simulink model "CessnaCitationCitationIIModel550_3DOF_control"  (R2020b)
settings: Solver=ode45  StartTime=0.0  StopTime=inf  FixedStep=1e-14  RelTol=1e-3
PreLoadFcn:
  | CessnaCitationData
  | datcom_data = datcomimport('Citation.out'); %Datcom data structures
  | datcom_data = FixDatcomData(datcom_data{3});
InitFcn:
  | CessnaCitationData
values from neighbouring files (symbols this model uses):
  gnd_alt = -1500    [CessnaCitationData.m]
  inertia = [19990.488, -0.000, 7138.962 ... (first row only)    [CessnaCitationData.m]
  initpos_e = [0 0 -1500]    [CessnaCitationData.m]
  initrotrates_e = [0 0 0]    [CessnaCitationData.m]
  initrpy_e = [0 0 0]    [CessnaCitationData.m]
  initvel_b = [85 0 0]    [CessnaCitationData.m]
  K = [-1.67126776797  253.63980268  1.10078856748  -2.4851948262  39.0629348129; 35.3806265678  -3943.84542644  -7.5960479952  17.7911501004  203.328962985]    [state_feedback_gain.mat]
  mass = 3175    [CessnaCitationData.m]
  max_thrust = 1134    [CessnaCitationData.m]
  wind_angle_rates = [0 0 0]    [CessnaCitationData.m]
undefined symbols (not defined in the file or in its folder): Earth, WGS84
libraries: aerolibtransform2 x5, aerolibasang x4, aerolibadyn x2, aerolibanim x1, aerolibwind2 x1, aerolibatmos2 x1, shared3dof x1, sharedtransform x1, simulink_extras x1
settings Model: Creator=pasquale  LastModifiedBy=pasquale
settings DataIOCC: ExternalInput=getinputstruct(op_trim1)  InitialState=getstatestruct(op_trim1)

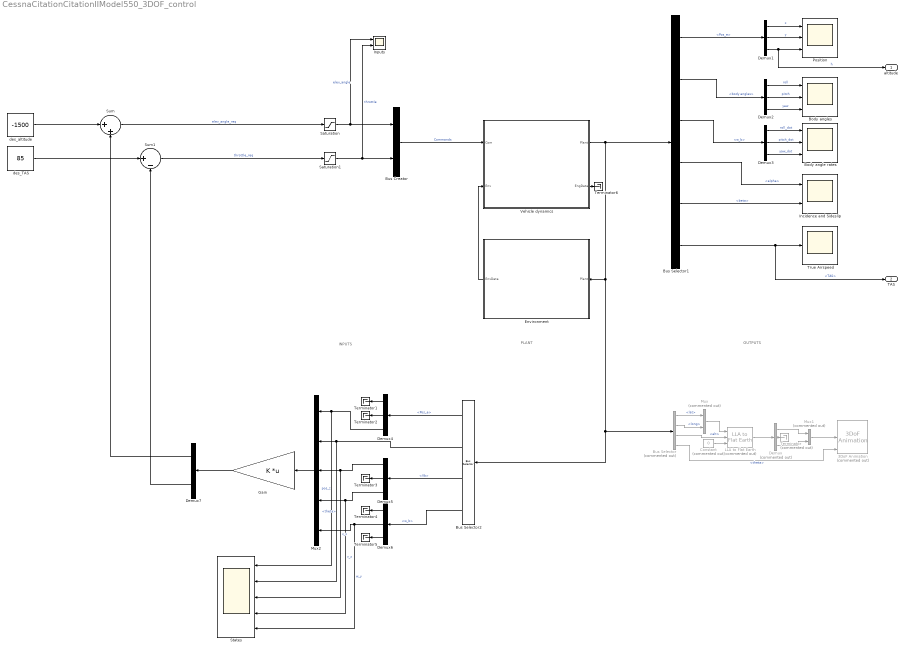
== system CessnaCitationCitationIIModel550_3DOF_control ==
  note: OUTPUTS
  note: PLANT
  note: INPUTS
  3DoF Animation : aerolibanim/3DoF Animation  Commented=on  u1=[0 5000 -2000 2000 -5050 -3050]  u2=0.05  u3=1.0  u5=Fixed position  u6=[2000 500 -3150]  u7=10  u8=on
      settings: SourceProductBaseCode=AE
  Body angle rates : Scope  NumInputPorts=3
  Body angles : Scope  NumInputPorts=3
  Bus Creator : BusCreator  Inputs=2
  Bus Selector : BusSelector  Commented=on  OutputSignals=lat,long,alt,body angles.theta
  Bus Selector1 : BusSelector  OutputSignals=Pos_e,body angles,w_b,alpha,beta,TAS
  Bus Selector2 : BusSelector  OutputSignals=Pos_e,body angles.theta,Vb,w_b
  Constant : Constant  Commented=on  Value=0
  Demux : Demux  Commented=on  Outputs=3
  Demux{1..6} (6 alike) : Demux  Outputs=3
  Demux7 : Demux  Outputs=2
  Environment : Subsystem
      mask Display: image('521928855-56a132c45f9b58b7d0bcf732-1.jpg'); % Use "Edit Image" on toolstrip to change.
  Gain : Gain  Gain=K  Multiplication=Matrix(K*u)
  Incidence and Sideslip : Scope  NumInputPorts=2
  Inputs : Scope  NumInputPorts=2
  LLA to Flat Earth : aerolibtransform2/LLA to Flat Earth  Commented=on  units=Metric (MKS)  ptype=Earth (WGS84)  F=1/298.257223563  R=6378137  refPosPort=off  LL0=[0 10]  psi=0
      settings: SourceProductBaseCode=AE
  Mux : Mux  Commented=on  Inputs=2
  Mux1 : Mux  Commented=on  Inputs=2
  Mux2 : Mux  Inputs=5
  Position : Scope  NumInputPorts=3
  Saturation : Saturate  UpperLimit=20  LowerLimit=-20
  Saturation1 : Saturate  UpperLimit=10000  LowerLimit=0
  States : Scope  NumInputPorts=5
  Sum : Sum  Inputs=|++
  Sum1 : Sum  Inputs=|+-
  Terminator : Terminator  Commented=on
  Terminator{1..6} (6 alike) : Terminator
  True Airspeed : Scope
  Vehicle dynamics : Subsystem
      mask Display: image('Cessna-Citation-II-IISP-S.jpg'); % Use "Edit Image" on toolstrip to change.
  des_TAS : Constant  Value=85
  des_altitude : Constant  Value=-1500
  altitude : Outport
  TAS : Outport  Port=2
  wires:
  Environment/1(EnvData) -> Vehicle dynamics/2(Env)
  Constant/1 -> LLA to Flat Earth/3
  Bus Selector/1 -> Mux/1  "<lat>"
  Bus Selector/2 -> Mux/2  "<long>"
  Mux/1 -> LLA to Flat Earth/1
  Bus Selector/3 -> LLA to Flat Earth/2  "<alt>"
  Bus Selector/4 -> 3DoF Animation/3  "<theta>"
  LLA to Flat Earth/1 -> Demux/1
  Demux/1 -> Mux1/1
  Demux/3 -> Mux1/2
  Demux/2 -> Terminator/1
  Mux1/1 -> 3DoF Animation/2
  Vehicle dynamics/1(Plant) -> Environment/1(Plant), Bus Selector2/1, Bus Selector/1, Bus Selector1/1
  Bus Creator/1 -> Vehicle dynamics/1(Com)  "Commands"
  Bus Selector1/1 -> Demux1/1  "<Pos_e>"
  Demux1/1 -> Position/1  "x"
  Demux1/2 -> Position/2  "y"
  Demux1/3 -> Position/3, altitude/1  "h"
  Bus Selector1/2 -> Demux2/1  "<body angles>"
  Demux2/1 -> Body angles/1  "roll"
  Demux2/2 -> Body angles/2  "pitch"
  Demux2/3 -> Body angles/3  "yaw"
  Bus Selector1/3 -> Demux3/1  "<w_b>"
  Demux3/1 -> Body angle rates/1  "roll_dot"
  Demux3/2 -> Body angle rates/2  "pitch_dot"
  Demux3/3 -> Body angle rates/3  "yaw_dot"
  Bus Selector1/4 -> Incidence and Sideslip/1  "<alpha>"
  Bus Selector1/5 -> Incidence and Sideslip/2  "<beta>"
  Bus Selector1/6 -> TAS/1, True Airspeed/1  "<TAS>"
  Bus Selector2/1 -> Demux4/1  "<Pos_e>"
  Bus Selector2/2 -> States/2, Mux2/2  "<theta>"
  Bus Selector2/3 -> Demux5/1  "<Vb>"
  Bus Selector2/4 -> Demux6/1  "<w_b>"
  Demux4/3 -> States/1, Mux2/1  "pos_z"
  Demux5/1 -> States/3, Mux2/3  "v_x"
  Demux6/2 -> States/5, Mux2/5  "w_y"
  Demux4/1 -> Terminator1/1
  Demux6/3 -> Terminator5/1
  Demux6/1 -> Terminator4/1
  Demux5/2 -> Terminator3/1
  Demux4/2 -> Terminator2/1
  Demux7/1 -> Sum/2
  Demux7/2 -> Sum1/2
  des_altitude/1 -> Sum/1
  des_TAS/1 -> Sum1/1
  Sum/1 -> Saturation/1  "elev_angle_req"
  Sum1/1 -> Saturation1/1  "throttle_req"
  Vehicle dynamics/2(EngData) -> Terminator6/1
  Saturation/1 -> Inputs/1, Bus Creator/1  "elev_angle"
  Saturation1/1 -> Inputs/2, Bus Creator/2  "throttle"
  Demux5/3 -> States/4, Mux2/4  "v_z"
  Mux2/1 -> Gain/1
  Gain/1 -> Demux7/1

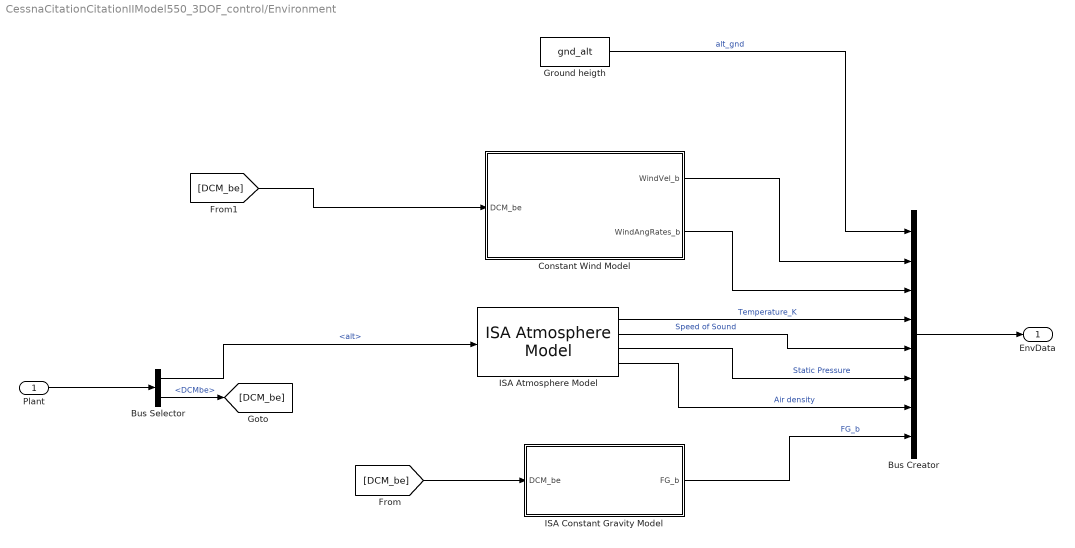
== system CessnaCitationCitationIIModel550_3DOF_control/Environment ==
  Plant : Inport
  Bus Creator : BusCreator  Inputs=8
  Bus Selector : BusSelector  OutputSignals=alt,DCMbe
  Constant Wind Model : Subsystem
  Ground heigth : Constant  Value=gnd_alt
  ISA Atmosphere Model : aerolibatmos2/ISA Atmosphere Model  custom=off  g=9.80665  gamma=1.4  R=287.0531  L=0.0065  h_trop=11000  h_strat=20000  rho0=1.225  P0=101325  T0=288.15  h0=0
  ISA Constant Gravity Model : Subsystem
  EnvData : Outport
  wires:
  Plant/1 -> Bus Selector/1
  Bus Selector/1 -> ISA Atmosphere Model/1  "<alt>"
  Bus Creator/1 -> EnvData/1
  ISA Atmosphere Model/4 -> Bus Creator/7  "Air density"
  ISA Atmosphere Model/3 -> Bus Creator/6  "Static Pressure"
  ISA Atmosphere Model/2 -> Bus Creator/5  "Speed of Sound"
  ISA Atmosphere Model/1 -> Bus Creator/4  "Temperature_K"
  Bus Selector/2 -> [DCM_be]  "<DCMbe>"
  [DCM_be] -> Constant Wind Model/1(DCM_be)
  Constant Wind Model/1(WindVel_b) -> Bus Creator/2
  Constant Wind Model/2(WindAngRates_b) -> Bus Creator/3
  ISA Constant Gravity Model/1(FG_b) -> Bus Creator/8  "FG_b"
  [DCM_be] -> ISA Constant Gravity Model/1(DCM_be)
  Ground heigth/1 -> Bus Creator/1  "alt_gnd"

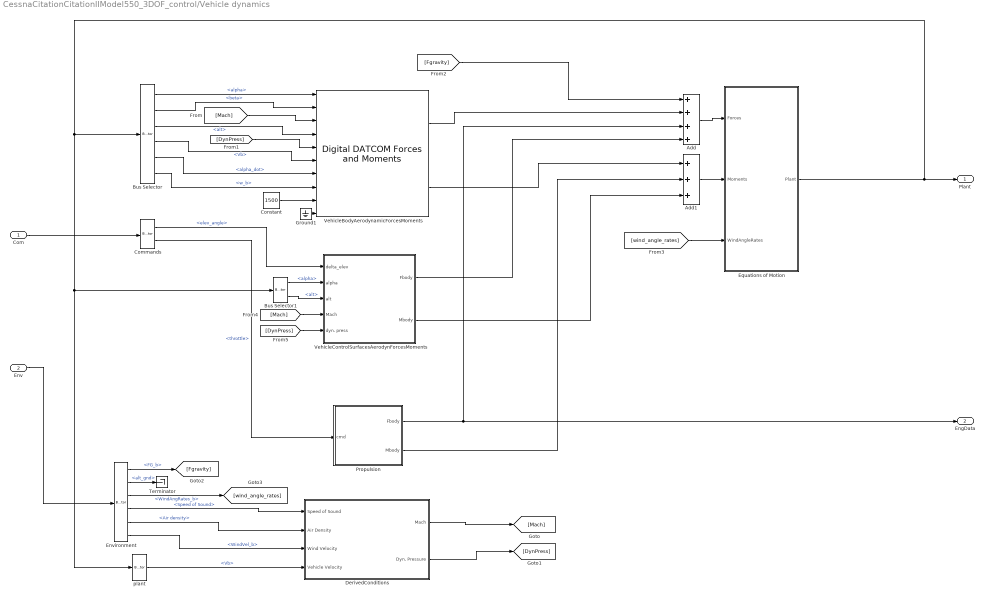
== system CessnaCitationCitationIIModel550_3DOF_control/Vehicle dynamics ==
  Com : Inport
  Env : Inport  Port=2
  Add : Sum  Inputs=++++
  Add1 : Sum  Inputs=+++
  Bus Selector : BusSelector  OutputSignals=alpha,beta,alt,Vb,alpha_dot,w_b
  Bus Selector1 : BusSelector  OutputSignals=alpha,alt
  Commands : BusSelector  OutputSignals=elev_angle,throttle
  Constant : Constant  Value=1500
  DerivedConditions : Subsystem
  Environment : BusSelector  OutputSignals=FG_b,alt_gnd,WindAngRates_b,Speed of Sound,Air density,WindVel_b
  Equations of Motion : Subsystem
  Ground1 : Ground
  Propulsion : Subsystem
  Terminator : Terminator
  VehicleBodyAerodynamicForcesMoments : aerolibadyn/Digital DATCOM Forces and Moments  units=Metric (MKS)  dcase=datcom_data  fmode=Body  buildno=0  imethod=Linear  emethod=Linear  rmethod=Linear Extrapolation  action=None
      settings: SourceProductBaseCode=AE
  VehicleControlSurfacesAerodynForcesMoments : Subsystem
  plant : BusSelector  OutputSignals=Vb
  Plant : Outport
  EngData : Outport  Port=2
  wires:
  Propulsion/1(Fbody) -> Add/3, EngData/1
  DerivedConditions/2(Dyn. Pressure) -> [DynPress]
  DerivedConditions/1(Mach) -> [Mach]
  [Mach] -> VehicleBodyAerodynamicForcesMoments/3
  [DynPress] -> VehicleBodyAerodynamicForcesMoments/5
  Bus Selector/2 -> VehicleBodyAerodynamicForcesMoments/2  "<beta>"
  Bus Selector/3 -> VehicleBodyAerodynamicForcesMoments/4  "<alt>"
  Bus Selector/4 -> VehicleBodyAerodynamicForcesMoments/6  "<Vb>"
  Bus Selector/6 -> VehicleBodyAerodynamicForcesMoments/8  "<w_b>"
  plant/1 -> DerivedConditions/4(Vehicle Velocity)  "<Vb>"
  Equations of Motion/1(Plant) -> plant/1, Bus Selector1/1, Bus Selector/1, Plant/1
  Env/1 -> Environment/1
  Com/1 -> Commands/1
  Environment/6 -> DerivedConditions/3(Wind Velocity)  "<WindVel_b>"
  Environment/5 -> DerivedConditions/2(Air Density)  "<Air density>"
  Environment/4 -> DerivedConditions/1(Speed of Sound)  "<Speed of Sound>"
  Commands/2 -> Propulsion/1(cmd)  "<throttle>"
  Bus Selector/1 -> VehicleBodyAerodynamicForcesMoments/1  "<alpha>"
  Bus Selector/5 -> VehicleBodyAerodynamicForcesMoments/7  "<alpha_dot>"
  Commands/1 -> VehicleControlSurfacesAerodynForcesMoments/1(delta_elev)  "<elev_angle>"
  Environment/1 -> [Fgravity]  "<FG_b>"
  Environment/3 -> [wind_angle_rates]  "<WindAngRates_b>"
  [wind_angle_rates] -> Equations of Motion/3(WindAngleRates)
  [Fgravity] -> Add/1
  VehicleBodyAerodynamicForcesMoments/1 -> Add/2
  VehicleBodyAerodynamicForcesMoments/2 -> Add1/1
  Propulsion/2(Mbody) -> Add1/2
  Add/1 -> Equations of Motion/1(Forces)
  Add1/1 -> Equations of Motion/2(Moments)
  VehicleControlSurfacesAerodynForcesMoments/1(Fbody) -> Add/4
  VehicleControlSurfacesAerodynForcesMoments/2(Mbody) -> Add1/3
  Bus Selector1/1 -> VehicleControlSurfacesAerodynForcesMoments/2(alpha)  "<alpha>"
  Bus Selector1/2 -> VehicleControlSurfacesAerodynForcesMoments/3(alt)  "<alt>"
  [DynPress] -> VehicleControlSurfacesAerodynForcesMoments/5(dyn. press)
  [Mach] -> VehicleControlSurfacesAerodynForcesMoments/4(Mach)
  Constant/1 -> VehicleBodyAerodynamicForcesMoments/9
  Ground1/1 -> VehicleBodyAerodynamicForcesMoments/10
  Environment/2 -> Terminator/1  "<alt_gnd>"

== system CessnaCitationCitationIIModel550_3DOF_control/Environment/Constant Wind Model ==
  DCM_be : Inport
  Horizontal Wind Model : aerolibwind2/Horizontal Wind Model  units=Metric (MKS)  Vw_source=Internal  Vwind=wind_speed  W_source=Internal  Wdeg=wind_dir
      settings: SourceProductBaseCode=AE
  Product2 : Product  Multiplication=Matrix(*)
  Wind_ang_rates : Constant  Value=wind_angle_rates
  WindVel_b : Outport
  WindAngRates_b : Outport  Port=2
  wires:
  DCM_be/1 -> Horizontal Wind Model/1, Product2/1
  Horizontal Wind Model/1 -> WindVel_b/1  "WindVel_b"
  Wind_ang_rates/1 -> Product2/2
  Product2/1 -> WindAngRates_b/1  "WindAngRates_b"

== system CessnaCitationCitationIIModel550_3DOF_control/Environment/ISA Constant Gravity Model ==
  DCM_be : Inport
  Gain : Gain  Gain=[0 0 mass]
  ISA constant gravity : Constant  Value=9.80665
  Product : Product  Multiplication=Matrix(*)
  FG_b : Outport
  wires:
  ISA constant gravity/1 -> Gain/1
  Gain/1 -> Product/2  "Fg in flat earth axis"
  DCM_be/1 -> Product/1
  Product/1 -> FG_b/1  "FG_b"

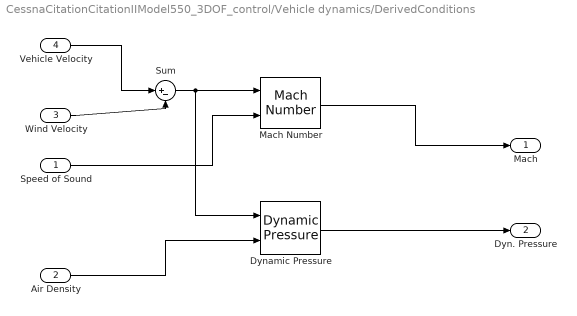
== system CessnaCitationCitationIIModel550_3DOF_control/Vehicle dynamics/DerivedConditions ==
  Speed of Sound : Inport
  Air Density : Inport  Port=2
  Wind Velocity : Inport  Port=3
  Vehicle Velocity : Inport  Port=4
  Dynamic Pressure : aerolibasang/Dynamic Pressure
  Mach Number : aerolibasang/Mach Number
      settings: SourceProductBaseCode=AE
  Sum : Sum  Inputs=|+-
  Mach : Outport
  Dyn. Pressure : Outport  Port=2
  wires:
  Vehicle Velocity/1 -> Sum/1
  Wind Velocity/1 -> Sum/2
  Sum/1 -> Dynamic Pressure/1, Mach Number/1
  Speed of Sound/1 -> Mach Number/2
  Mach Number/1 -> Mach/1
  Dynamic Pressure/1 -> Dyn. Pressure/1
  Air Density/1 -> Dynamic Pressure/2

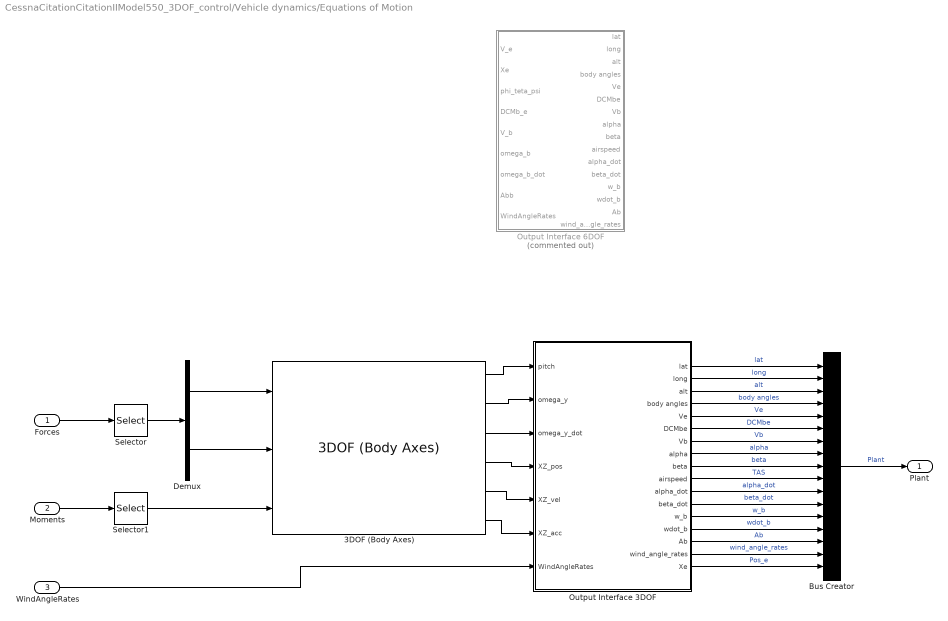
== system CessnaCitationCitationIIModel550_3DOF_control/Vehicle dynamics/Equations of Motion ==
  Forces : Inport
  Moments : Inport  Port=2
  WindAngleRates : Inport  Port=3
  3DOF (Body Axes) : shared3dof/3DOF (Body Axes)  units=Metric (MKS)  mtype=Fixed  v_ini=initvel_b(1)  theta_ini=initrpy_e(2)  alpha_ini=0  pos_ini=[initpos_e(1) initpos_e(3)]  q_ini=initrotrates_e(2)  mass=mass  mass_e=0.5  mass_f=3.0  Iyy=inertia(2,2)  Iyy_e=0.5  Iyy_f=3.0  g_in=Internal  g=0  vre_flag=on  abi_flag=off  aMode=0  vel_statename=''  theta_statename=''  pos_statename=''  q_statename=''  mass_statename=''
      settings: SourceProductBaseCode=AE,PW,MT,UV,VE,VP
  Bus Creator : BusCreator  Inputs=17
  Demux : Demux  Outputs=2
  Output Interface 3DOF : Subsystem
  Output Interface 6DOF : Subsystem  Commented=on
  Selector : Selector  InputPortWidth=3  IndexOptions=Index vector (dialog)  Indices=[1 3]  OutputSizes=1
  Selector1 : Selector  InputPortWidth=3  IndexOptions=Index vector (dialog)  Indices=[2]  OutputSizes=1
  Plant : Outport
  wires:
  Bus Creator/1 -> Plant/1  "Plant"
  Forces/1 -> Selector/1
  Demux/1 -> 3DOF (Body Axes)/1
  Demux/2 -> 3DOF (Body Axes)/2
  Selector/1 -> Demux/1
  Moments/1 -> Selector1/1
  Selector1/1 -> 3DOF (Body Axes)/3
  3DOF (Body Axes)/3 -> Output Interface 3DOF/3(omega_y_dot)
  3DOF (Body Axes)/1 -> Output Interface 3DOF/1(pitch)
  3DOF (Body Axes)/2 -> Output Interface 3DOF/2(omega_y)
  3DOF (Body Axes)/4 -> Output Interface 3DOF/4(XZ_pos)
  3DOF (Body Axes)/5 -> Output Interface 3DOF/5(XZ_vel)
  3DOF (Body Axes)/6 -> Output Interface 3DOF/6(XZ_acc)
  Output Interface 3DOF/1(lat) -> Bus Creator/1  "lat"
  Output Interface 3DOF/2(long) -> Bus Creator/2  "long"
  Output Interface 3DOF/3(alt) -> Bus Creator/3  "alt"
  Output Interface 3DOF/4(body angles) -> Bus Creator/4  "body angles"
  Output Interface 3DOF/5(Ve) -> Bus Creator/5  "Ve"
  Output Interface 3DOF/6(DCMbe) -> Bus Creator/6  "DCMbe"
  Output Interface 3DOF/7(Vb) -> Bus Creator/7  "Vb"
  Output Interface 3DOF/8(alpha) -> Bus Creator/8  "alpha"
  Output Interface 3DOF/9(beta) -> Bus Creator/9  "beta"
  Output Interface 3DOF/10(airspeed) -> Bus Creator/10  "TAS"
  Output Interface 3DOF/11(alpha_dot) -> Bus Creator/11  "alpha_dot"
  Output Interface 3DOF/12(beta_dot) -> Bus Creator/12  "beta_dot"
  Output Interface 3DOF/13(w_b) -> Bus Creator/13  "w_b"
  Output Interface 3DOF/14(wdot_b) -> Bus Creator/14  "wdot_b"
  Output Interface 3DOF/15(Ab) -> Bus Creator/15  "Ab"
  Output Interface 3DOF/16(wind_angle_rates) -> Bus Creator/16  "wind_angle_rates"
  WindAngleRates/1 -> Output Interface 3DOF/7(WindAngleRates)
  Output Interface 3DOF/17(Xe) -> Bus Creator/17  "Pos_e"

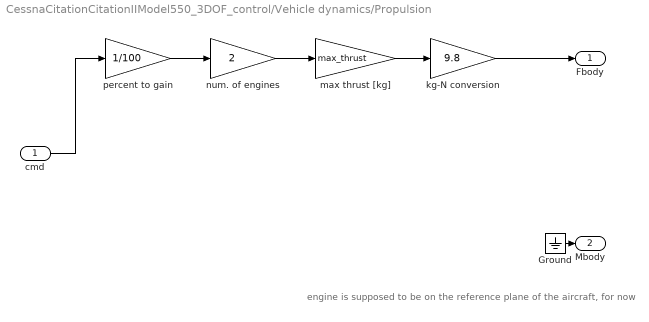
== system CessnaCitationCitationIIModel550_3DOF_control/Vehicle dynamics/Propulsion ==
  note: engine is supposed to be on the reference plane of the aircraft, for now
  cmd : Inport
  Ground : Ground
  kg-N conversion : Gain  Gain=9.8
  max thrust [kg] : Gain  Gain=max_thrust
  num. of engines : Gain  Gain=2
  percent to gain : Gain  Gain=1/100
  Fbody : Outport
  Mbody : Outport  Port=2
  wires:
  percent to gain/1 -> num. of engines/1
  cmd/1 -> percent to gain/1
  max thrust [kg]/1 -> kg-N conversion/1
  kg-N conversion/1 -> Fbody/1
  Ground/1 -> Mbody/1
  num. of engines/1 -> max thrust [kg]/1

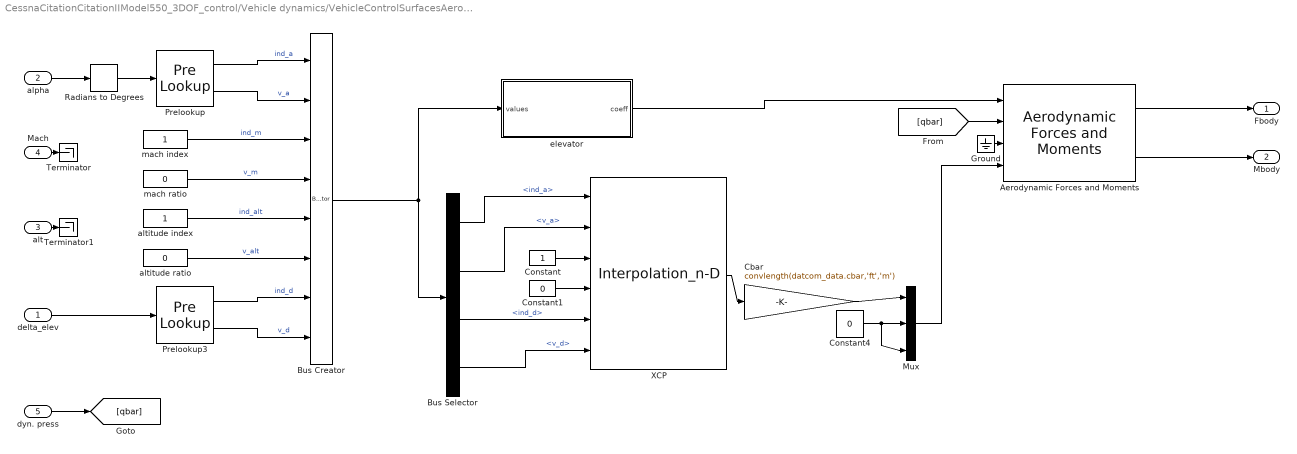
== system CessnaCitationCitationIIModel550_3DOF_control/Vehicle dynamics/VehicleControlSurfacesAerodynForcesMoments ==
  delta_elev : Inport
  alpha : Inport  Port=2
  alt : Inport  Port=3
  Mach : Inport  Port=4
  dyn. press : Inport  Port=5
  "Aerodynamic Forces and Moments " : aerolibadyn/Aerodynamic Forces and Moments   inputAxes=Body  outputForceAxes=Body  outputMomentAxes=Body  S=convlength(datcom_data.sref,'ft','m')  b=convlength(datcom_data.blref,'ft','m')  cbar=convlength(datcom_data.cbar,'ft','m')
  Bus Creator : BusCreator  Inputs=8
  Bus Selector : BusSelector  OutputSignals=ind_a,v_a,ind_d,v_d
  Cbar : Gain  Gain=convlength(datcom_data.cbar,'ft','m')
  Constant : Constant
  Constant1 : Constant  Value=0
  Constant4 : Constant  Value=0
  Ground : Ground
  Mux : Mux  Inputs=3
  Prelookup : PreLookup  BreakpointsData=datcom_data.alpha  ExtrapMethod=Linear
  Prelookup3 : PreLookup  BreakpointsData=datcom_data.delta  ExtrapMethod=Linear
  Radians to Degrees : simulink_extras/Transformations/Radians to Degrees
  Terminator : Terminator
  Terminator1 : Terminator
  XCP : Interpolation_n-D  NumberOfTableDimensions=3  Table=reshape(datcom_data.xcp, [20 2 9]);  InternalRulePriority=Speed
      settings: InputPortMap=u0,u1,u2,u3,u4,u5
  altitude index : Constant
  altitude ratio : Constant  Value=0
  elevator : Subsystem
  mach index : Constant
  mach ratio : Constant  Value=0
  Fbody : Outport
  Mbody : Outport  Port=2
  wires:
  alpha/1 -> Radians to Degrees/1
  Radians to Degrees/1 -> Prelookup/1
  delta_elev/1 -> Prelookup3/1
  Prelookup/1 -> Bus Creator/1  "ind_a"
  Prelookup/2 -> Bus Creator/2  "v_a"
  Prelookup3/1 -> Bus Creator/7  "ind_d"
  Prelookup3/2 -> Bus Creator/8  "v_d"
  Bus Creator/1 -> elevator/1(values), Bus Selector/1
  Mach/1 -> Terminator/1
  alt/1 -> Terminator1/1
  mach index/1 -> Bus Creator/3  "ind_m"
  mach ratio/1 -> Bus Creator/4  "v_m"
  altitude index/1 -> Bus Creator/5  "ind_alt"
  altitude ratio/1 -> Bus Creator/6  "v_alt"
  dyn. press/1 -> [qbar]
  [qbar] -> "Aerodynamic Forces and Moments "/2
  Ground/1 -> "Aerodynamic Forces and Moments "/3
  elevator/1(coeff) -> "Aerodynamic Forces and Moments "/1
  Bus Selector/1 -> XCP/1  "<ind_a>"
  Bus Selector/2 -> XCP/2  "<v_a>"
  Constant1/1 -> XCP/4
  Constant/1 -> XCP/3
  Bus Selector/3 -> XCP/5  "<ind_d>"
  Bus Selector/4 -> XCP/6  "<v_d>"
  XCP/1 -> Cbar/1
  Constant4/1 -> Mux/3, Mux/2
  Mux/1 -> "Aerodynamic Forces and Moments "/4
  "Aerodynamic Forces and Moments "/1 -> Fbody/1
  "Aerodynamic Forces and Moments "/2 -> Mbody/1
  Cbar/1 -> Mux/1

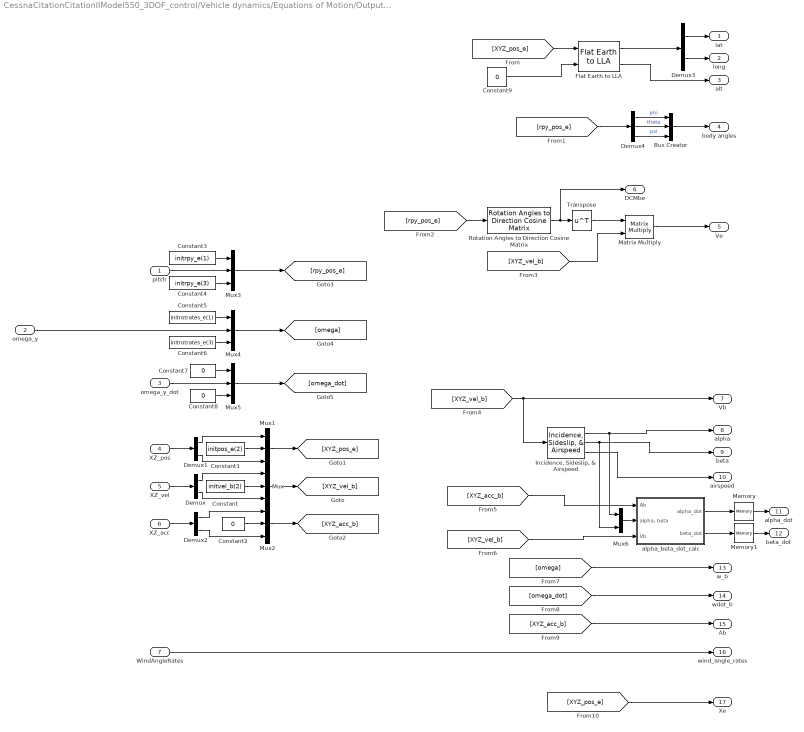
== system CessnaCitationCitationIIModel550_3DOF_control/Vehicle dynamics/Equations of Motion/Output Interface 3DOF ==
  pitch : Inport
  omega_y : Inport  Port=2
  omega_y_dot : Inport  Port=3
  XZ_pos : Inport  Port=4
  XZ_vel : Inport  Port=5
  XZ_acc : Inport  Port=6
  WindAngleRates : Inport  Port=7
  Bus Creator : BusCreator  Inputs=3
  Constant : Constant  Value=initvel_b(2)
  Constant1 : Constant  Value=initpos_e(2)
  Constant{2,7..9} (4 alike) : Constant  Value=0
  Constant3 : Constant  Value=initrpy_e(1)
  Constant4 : Constant  Value=initrpy_e(3)
  Constant5 : Constant  Value=initrotrates_e(1)
  Constant6 : Constant  Value=initrotrates_e(3)
  Demux{,1..3} (4 alike) : Demux  Outputs=2
  Demux4 : Demux  Outputs=3
  Flat Earth to LLA : aerolibtransform2/Flat Earth to LLA  units=Metric (MKS)  ptype=Earth (WGS84)  F=1/298.257223563  R=6378137  refPosPort=off  LL0=[0 10]  psi=0
  "Incidence, Sideslip, & Airspeed" : aerolibasang/Incidence, Sideslip, & Airspeed
  Matrix Multiply : Product  Multiplication=Matrix(*)
  Memory : Memory
  Memory1 : Memory
  Mux{,1..5} (6 alike) : Mux  Inputs=3
  Mux6 : Mux  Inputs=2
  Rotation Angles to Direction Cosine Matrix : sharedtransform/Rotation Angles to Direction Cosine Matrix  rotationOrder=ZYX  aMode=aMode
      settings: SourceProductBaseCode=AE,PW,MT,UV,VE,VP
  Transpose : Math  Operator=transpose  SaturateOnIntegerOverflow=on
  alpha_beta_dot_calc : Subsystem
  lat : Outport
  long : Outport  Port=2
  alt : Outport  Port=3
  body angles : Outport  Port=4
  Ve : Outport  Port=5
  DCMbe : Outport  Port=6
  Vb : Outport  Port=7
  alpha : Outport  Port=8
  beta : Outport  Port=9
  airspeed : Outport  Port=10
  alpha_dot : Outport  Port=11
  beta_dot : Outport  Port=12
  w_b : Outport  Port=13
  wdot_b : Outport  Port=14
  Ab : Outport  Port=15
  wind_angle_rates : Outport  Port=16
  Xe : Outport  Port=17
  wires:
  WindAngleRates/1 -> wind_angle_rates/1
  XZ_vel/1 -> Demux/1
  Constant/1 -> Mux/2
  Demux/1 -> Mux/1
  Demux/2 -> Mux/3
  Mux/1 -> [XYZ_vel_b]
  Mux1/1 -> [XYZ_pos_e]
  Demux1/2 -> Mux1/3
  Demux1/1 -> Mux1/1
  Constant1/1 -> Mux1/2
  XZ_pos/1 -> Demux1/1
  Constant2/1 -> Mux2/2
  Demux2/2 -> Mux2/3
  XZ_acc/1 -> Demux2/1
  Mux2/1 -> [XYZ_acc_b]
  Demux2/1 -> Mux2/1
  pitch/1 -> Mux3/2
  Constant3/1 -> Mux3/1
  Constant4/1 -> Mux3/3
  Mux3/1 -> [rpy_pos_e]
  Mux4/1 -> [omega]
  Constant6/1 -> Mux4/3
  Constant5/1 -> Mux4/1
  omega_y/1 -> Mux4/2
  omega_y_dot/1 -> Mux5/2
  Constant7/1 -> Mux5/1
  Constant8/1 -> Mux5/3
  Mux5/1 -> [omega_dot]
  Demux3/1 -> lat/1
  Demux3/2 -> long/1
  Flat Earth to LLA/1 -> Demux3/1
  Flat Earth to LLA/2 -> alt/1
  [XYZ_pos_e] -> Flat Earth to LLA/1
  Constant9/1 -> Flat Earth to LLA/2
  Demux4/2 -> Bus Creator/2  "theta"
  Demux4/1 -> Bus Creator/1  "phi"
  Demux4/3 -> Bus Creator/3  "psi"
  Bus Creator/1 -> body angles/1
  [rpy_pos_e] -> Demux4/1
  [rpy_pos_e] -> Rotation Angles to Direction Cosine Matrix/1
  Rotation Angles to Direction Cosine Matrix/1 -> DCMbe/1, Transpose/1
  Transpose/1 -> Matrix Multiply/1
  [XYZ_vel_b] -> Matrix Multiply/2
  Matrix Multiply/1 -> Ve/1
  [XYZ_vel_b] -> "Incidence, Sideslip, & Airspeed"/1, Vb/1
  "Incidence, Sideslip, & Airspeed"/1 -> Mux6/1, alpha/1
  "Incidence, Sideslip, & Airspeed"/2 -> Mux6/2, beta/1
  "Incidence, Sideslip, & Airspeed"/3 -> airspeed/1
  Memory/1 -> alpha_dot/1
  Memory1/1 -> beta_dot/1
  [omega] -> w_b/1
  [omega_dot] -> wdot_b/1
  [XYZ_acc_b] -> Ab/1
  alpha_beta_dot_calc/1(alpha_dot) -> Memory/1
  alpha_beta_dot_calc/2(beta_dot) -> Memory1/1
  Mux6/1 -> alpha_beta_dot_calc/2("alpha, beta")
  [XYZ_acc_b] -> alpha_beta_dot_calc/1(Ab)
  [XYZ_vel_b] -> alpha_beta_dot_calc/3(Vb)
  [XYZ_pos_e] -> Xe/1

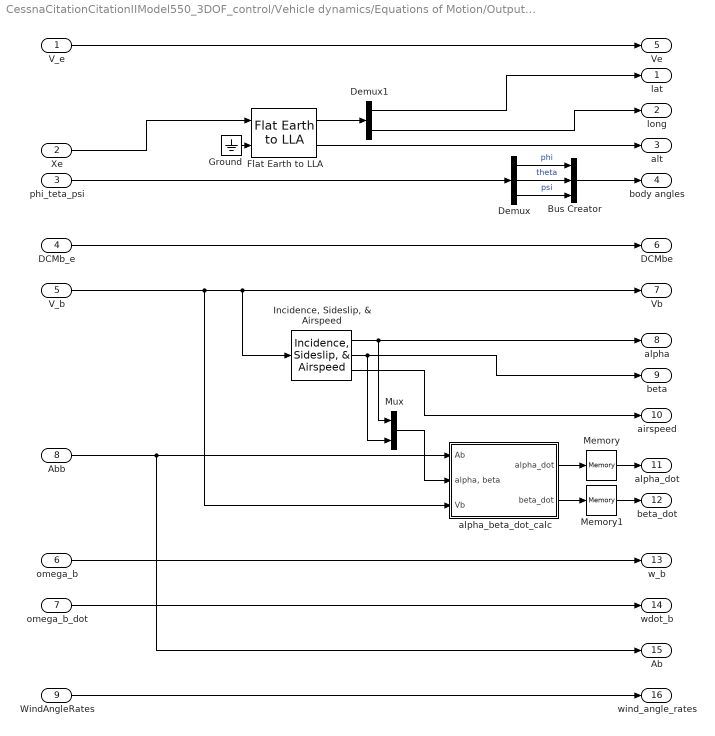
== system CessnaCitationCitationIIModel550_3DOF_control/Vehicle dynamics/Equations of Motion/Output Interface 6DOF ==
  V_e : Inport
  Xe : Inport  Port=2
  phi_teta_psi : Inport  Port=3
  DCMb_e : Inport  Port=4
  V_b : Inport  Port=5
  omega_b : Inport  Port=6
  omega_b_dot : Inport  Port=7
  Abb : Inport  Port=8
  WindAngleRates : Inport  Port=9
  Bus Creator : BusCreator  Inputs=3
  Demux : Demux  Outputs=3
  Demux1 : Demux  Outputs=2
  Flat Earth to LLA : aerolibtransform2/Flat Earth to LLA  units=Metric (MKS)  ptype=Earth (WGS84)  F=1/298.257223563  R=6378137  refPosPort=off  LL0=[0 10]  psi=0
  Ground : Ground
  "Incidence, Sideslip, & Airspeed" : aerolibasang/Incidence, Sideslip, & Airspeed
  Memory : Memory
  Memory1 : Memory
  Mux : Mux  Inputs=2
  alpha_beta_dot_calc : Subsystem
  lat : Outport
  long : Outport  Port=2
  alt : Outport  Port=3
  body angles : Outport  Port=4
  Ve : Outport  Port=5
  DCMbe : Outport  Port=6
  Vb : Outport  Port=7
  alpha : Outport  Port=8
  beta : Outport  Port=9
  airspeed : Outport  Port=10
  alpha_dot : Outport  Port=11
  beta_dot : Outport  Port=12
  w_b : Outport  Port=13
  wdot_b : Outport  Port=14
  Ab : Outport  Port=15
  wind_angle_rates : Outport  Port=16
  wires:
  Demux/2 -> Bus Creator/2  "theta"
  Ground/1 -> Flat Earth to LLA/2
  Demux/3 -> Bus Creator/3  "psi"
  Demux1/1 -> lat/1
  Flat Earth to LLA/2 -> alt/1
  Flat Earth to LLA/1 -> Demux1/1
  Demux1/2 -> long/1
  Demux/1 -> Bus Creator/1  "phi"
  Bus Creator/1 -> body angles/1
  phi_teta_psi/1 -> Demux/1
  Xe/1 -> Flat Earth to LLA/1
  DCMb_e/1 -> DCMbe/1
  V_b/1 -> alpha_beta_dot_calc/3(Vb), "Incidence, Sideslip, & Airspeed"/1, Vb/1
  "Incidence, Sideslip, & Airspeed"/1 -> Mux/1, alpha/1
  "Incidence, Sideslip, & Airspeed"/2 -> Mux/2, beta/1
  "Incidence, Sideslip, & Airspeed"/3 -> airspeed/1
  Abb/1 -> Ab/1, alpha_beta_dot_calc/1(Ab)
  Mux/1 -> alpha_beta_dot_calc/2("alpha, beta")
  V_e/1 -> Ve/1
  omega_b/1 -> w_b/1
  omega_b_dot/1 -> wdot_b/1
  WindAngleRates/1 -> wind_angle_rates/1
  alpha_beta_dot_calc/1(alpha_dot) -> Memory/1
  alpha_beta_dot_calc/2(beta_dot) -> Memory1/1
  Memory/1 -> alpha_dot/1
  Memory1/1 -> beta_dot/1

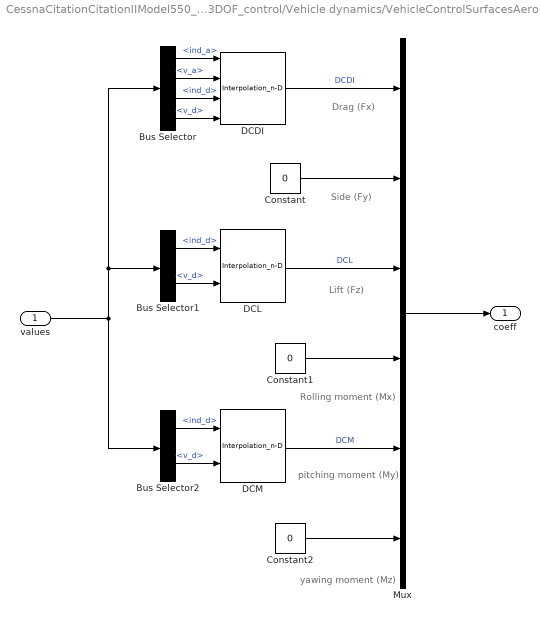
== system CessnaCitationCitationIIModel550_3DOF_control/Vehicle dynamics/VehicleControlSurfacesAerodynForcesMoments/elevator ==
  note: yawing moment (Mz)
  note: pitching moment (My)
  note: Rolling moment (Mx)
  note: Lift (Fz)
  note: Side (Fy)
  note: Drag (Fx)
  values : Inport
  Bus Selector : BusSelector  OutputSignals=ind_a,v_a,ind_d,v_d
  Bus Selector1 : BusSelector  OutputSignals=ind_d,v_d
  Bus Selector2 : BusSelector  OutputSignals=ind_d,v_d
  Constant : Constant  Value=0
  Constant1 : Constant  Value=0
  Constant2 : Constant  Value=0
  DCDI : Interpolation_n-D  Table=datcom_data.dcdi_sym  InternalRulePriority=Speed
  DCL : Interpolation_n-D  NumberOfTableDimensions=1  Table=datcom_data.dcl_sym  InternalRulePriority=Speed
      settings: InputPortMap=u0,u1
  DCM : Interpolation_n-D  NumberOfTableDimensions=1  Table=datcom_data.dcl_sym  InternalRulePriority=Speed
      settings: InputPortMap=u0,u1
  Mux : Mux  Inputs=6
  coeff : Outport
  wires:
  values/1 -> Bus Selector/1, Bus Selector1/1, Bus Selector2/1
  Bus Selector/1 -> DCDI/1  "<ind_a>"
  Bus Selector/2 -> DCDI/2  "<v_a>"
  Bus Selector/3 -> DCDI/3  "<ind_d>"
  Bus Selector/4 -> DCDI/4  "<v_d>"
  Bus Selector1/1 -> DCL/1  "<ind_d>"
  Bus Selector1/2 -> DCL/2  "<v_d>"
  Bus Selector2/1 -> DCM/1  "<ind_d>"
  Bus Selector2/2 -> DCM/2  "<v_d>"
  DCL/1 -> Mux/3  "DCL"
  DCDI/1 -> Mux/1  "DCDI"
  DCM/1 -> Mux/5  "DCM"
  Mux/1 -> coeff/1
  Constant/1 -> Mux/2
  Constant1/1 -> Mux/4
  Constant2/1 -> Mux/6

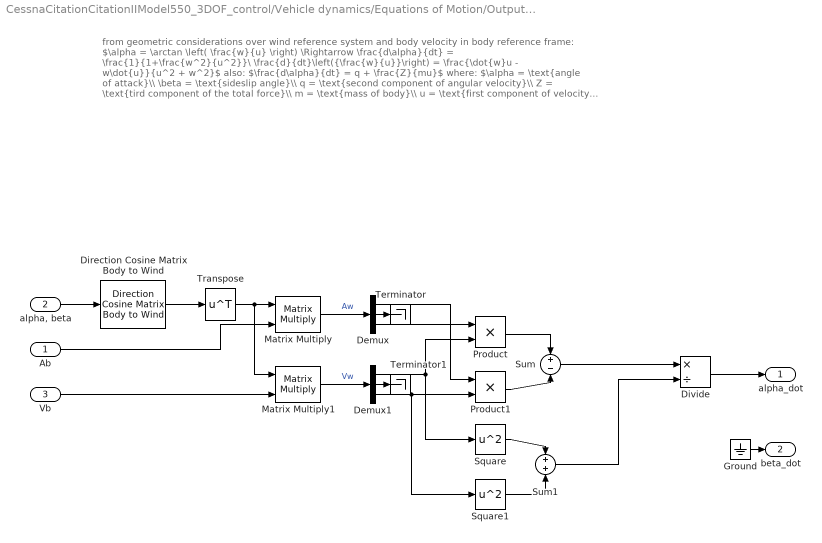
== system CessnaCitationCitationIIModel550_3DOF_control/Vehicle dynamics/Equations of Motion/Output Interface 3DOF/alpha_beta_dot_calc ==
  note: from geometric considerations over wind reference system and body velocity in body reference frame:
      | $\alpha = \arctan \left( \frac{w}{u} \right) \Rightarrow \frac{d\alpha}{dt} = \frac{1}{1+\frac{w^2}{u^2}}\ \frac{d}{dt}\left({\frac{w}{u}}\right) = \frac{\dot{w}u - w\dot{u}}{u^2 + w^2}$
      | also:
      | $\frac{d\alpha}{dt} = q + \frac{Z}{mu}$
      | where:
      | $\alpha = \text{angle of attack}\\ \beta = \text{sideslip angle}\\ q = \text{second component of angular velocity}\\ Z = \text{tird component of the total force}\\ m = \text{mass of body}\\ u = \text{first component of velocity in wind reference frame}\\ w = \text{third component of velocity in wind reference frame}$
      |
      | same can be done for $\dot{\beta}$
  Ab : Inport
  "alpha, beta" : Inport  Port=2
  Vb : Inport  Port=3
  Demux : Demux  Outputs=3
  Demux1 : Demux  Outputs=3
  Direction Cosine Matrix Body to Wind : aerolibtransform2/Direction Cosine Matrix Body to Wind
      settings: SourceProductBaseCode=AE
  Divide : Product  Inputs=*/
  Ground : Ground
  Matrix Multiply : Product  Multiplication=Matrix(*)
  Matrix Multiply1 : Product  Multiplication=Matrix(*)
  Product : Product
  Product1 : Product
  Square : Math  Operator=square  SaturateOnIntegerOverflow=on
  Square1 : Math  Operator=square  SaturateOnIntegerOverflow=on
  Sum : Sum  Inputs=+|-
  Sum1 : Sum  Inputs=+|+
  Terminator : Terminator
  Terminator1 : Terminator
  Transpose : Math  Operator=transpose  SaturateOnIntegerOverflow=on
  alpha_dot : Outport
  beta_dot : Outport  Port=2
  wires:
  "alpha, beta"/1 -> Direction Cosine Matrix Body to Wind/1
  Direction Cosine Matrix Body to Wind/1 -> Transpose/1
  Transpose/1 -> Matrix Multiply1/1, Matrix Multiply/1
  Ab/1 -> Matrix Multiply/2
  Vb/1 -> Matrix Multiply1/2
  Matrix Multiply1/1 -> Demux1/1  "Vw"
  Matrix Multiply/1 -> Demux/1  "Aw"
  Demux/3 -> Product/1
  Demux1/1 -> Square/1, Product/2
  Demux1/3 -> Square1/1, Product1/2
  Demux/1 -> Product1/1
  Product/1 -> Sum/1
  Product1/1 -> Sum/2
  Sum/1 -> Divide/1
  Square/1 -> Sum1/1
  Square1/1 -> Sum1/2
  Sum1/1 -> Divide/2
  Divide/1 -> alpha_dot/1
  Ground/1 -> beta_dot/1
  Demux/2 -> Terminator/1
  Demux1/2 -> Terminator1/1

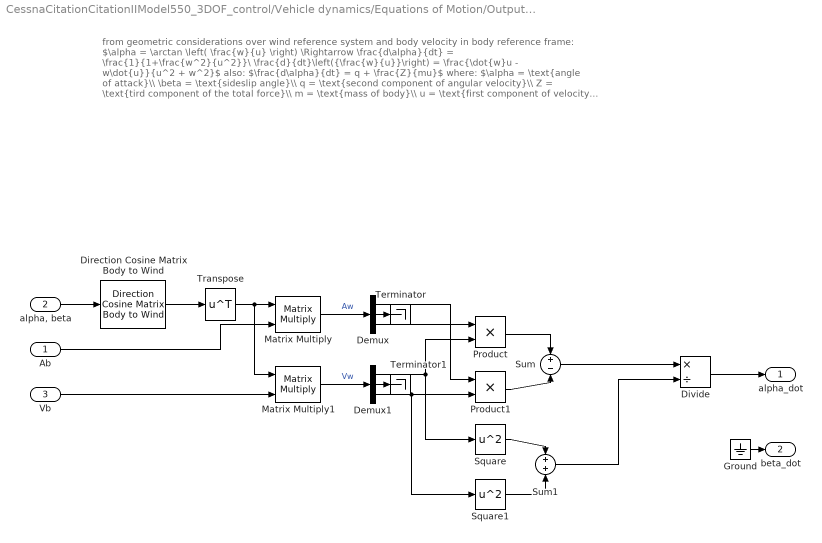
== system CessnaCitationCitationIIModel550_3DOF_control/Vehicle dynamics/Equations of Motion/Output Interface 6DOF/alpha_beta_dot_calc ==
  note: from geometric considerations over wind reference system and body velocity in body reference frame:
      | $\alpha = \arctan \left( \frac{w}{u} \right) \Rightarrow \frac{d\alpha}{dt} = \frac{1}{1+\frac{w^2}{u^2}}\ \frac{d}{dt}\left({\frac{w}{u}}\right) = \frac{\dot{w}u - w\dot{u}}{u^2 + w^2}$
      | also:
      | $\frac{d\alpha}{dt} = q + \frac{Z}{mu}$
      | where:
      | $\alpha = \text{angle of attack}\\ \beta = \text{sideslip angle}\\ q = \text{second component of angular velocity}\\ Z = \text{tird component of the total force}\\ m = \text{mass of body}\\ u = \text{first component of velocity in wind reference frame}\\ w = \text{third component of velocity in wind reference frame}$
      |
      | same can be done for $\dot{\beta}$
  Ab : Inport
  "alpha, beta" : Inport  Port=2
  Vb : Inport  Port=3
  Demux : Demux  Outputs=3
  Demux1 : Demux  Outputs=3
  Direction Cosine Matrix Body to Wind : aerolibtransform2/Direction Cosine Matrix Body to Wind
      settings: SourceProductBaseCode=AE
  Divide : Product  Inputs=*/
  Ground : Ground
  Matrix Multiply : Product  Multiplication=Matrix(*)
  Matrix Multiply1 : Product  Multiplication=Matrix(*)
  Product : Product
  Product1 : Product
  Square : Math  Operator=square  SaturateOnIntegerOverflow=on
  Square1 : Math  Operator=square  SaturateOnIntegerOverflow=on
  Sum : Sum  Inputs=+|-
  Sum1 : Sum  Inputs=+|+
  Terminator : Terminator
  Terminator1 : Terminator
  Transpose : Math  Operator=transpose  SaturateOnIntegerOverflow=on
  alpha_dot : Outport
  beta_dot : Outport  Port=2
  wires:
  "alpha, beta"/1 -> Direction Cosine Matrix Body to Wind/1
  Direction Cosine Matrix Body to Wind/1 -> Transpose/1
  Transpose/1 -> Matrix Multiply1/1, Matrix Multiply/1
  Ab/1 -> Matrix Multiply/2
  Vb/1 -> Matrix Multiply1/2
  Matrix Multiply1/1 -> Demux1/1  "Vw"
  Matrix Multiply/1 -> Demux/1  "Aw"
  Demux/3 -> Product/1
  Demux1/1 -> Square/1, Product/2
  Demux1/3 -> Square1/1, Product1/2
  Demux/1 -> Product1/1
  Product/1 -> Sum/1
  Product1/1 -> Sum/2
  Sum/1 -> Divide/1
  Square/1 -> Sum1/1
  Square1/1 -> Sum1/2
  Sum1/1 -> Divide/2
  Divide/1 -> alpha_dot/1
  Ground/1 -> beta_dot/1
  Demux/2 -> Terminator/1
  Demux1/2 -> Terminator1/1
